simulink model "modeldefinitiu4t"  (Simulink 7.4)
settings: Solver=ode45  StartTime=t0  StopTime=t1  MaxStep=1e-4
values from neighbouring files (symbols this model uses):
  Ap = 90e3*sqrt(2)/sqrt(3)    [parametres.m]
  E0 = 145e3    (= 145000)    [parametres.m]
  f = 50    [parametres.m]
  ida3 = 0    [parametres.m]
  ida4 = 0    [parametres.m]
  it = [0 0.2 0.200001 0.35 0.3500001 t1]    [parametres.m]
  iv = [0 0 100e6 100e6 0 0]    [parametres.m]
  K3 = 1/20    (= 0.05)    [parametres.m]
  K4 = K3    (= 0.05)    [parametres.m]
  Ki = rl/tau    (= 1140.8)    [parametres.m]
  Kp = Ll/tau    (= 93)    [parametres.m]
  L1 = 0.005    [parametres.m]
  L2 = 0.0025    [parametres.m]
  L3 = 0.004    [parametres.m]
  Lac = 30e-3    (= 0.03)    [parametres.m]
  Ll = Lac    (= 0.03)    [parametres.m]
  Lx = 0.052*0.669    (= 0.034788)    [parametres.m]
  R1 = 0.5    [parametres.m]
  R2 = 0.25    [parametres.m]
  R3 = 0.4    [parametres.m]
  Rac = 3.68/10    (= 0.368)    [parametres.m]
  Rx = 4.8*0.669    (= 3.2112)    [parametres.m]
  sc = 0    [parametres.m]
  T = 1/12e3    (= 8.33333333333e-05)    [parametres.m]
undefined symbols (not defined in the file or in its folder): DiscIntNeverNeededParam
libraries: powerlib x62
(part 2 of 2)

== system modeldefinitiu4t/Subsystem5/Càlcul de consignes ==
  note: P
  vzq3 : Inport
  E3 : Inport  Port=2
  Constant : Constant  Value=E0  OutDataType=fixdt(1, 16)  OutScaling=2^0
  Divide1 : Product  Inputs=*/  OutDataType=fixdt(1, 16)  OutScaling=2^-10
  Gain : Gain  Gain=K3  ParameterDataType=fixdt(1, 16)  ParameterScaling=2^0  OutDataType=fixdt(1, 16)  OutScaling=2^0
  Gain1 : Gain  Gain=2/3  ParameterDataType=fixdt(1, 16)  ParameterScaling=2^0  OutDataType=fixdt(1, 16)  OutScaling=2^0
  Gain2 : Gain  ParameterDataType=fixdt(1, 16)  ParameterScaling=2^0  OutDataType=fixdt(1, 16)  OutScaling=2^0  SampleTime=T
  Gain6 : Gain  ParameterDataType=fixdt(1, 16)  ParameterScaling=2^0  OutDataType=fixdt(1, 16)  OutScaling=2^0  SampleTime=T
  Gain7 : Gain  ParameterDataType=fixdt(1, 16)  ParameterScaling=2^0  OutDataType=fixdt(1, 16)  OutScaling=2^0  SampleTime=T
  Product : Product  OutDataType=fixdt(1, 16)  OutScaling=2^0  RndMeth=Zero
  Sum : Sum  Inputs=|+-  OutDataType=fixdt(1, 16)  OutScaling=2^0
  To Workspace3 : ToWorkspace  VariableName=Eref  SampleTime=-1  SaveFormat=Array
  iqa3 : Outport
  wires:
  Constant/1 -> Gain7/1
  Sum/1 -> Gain/1
  Product/1 -> Gain1/1
  Gain/1 -> Product/2
  Gain6/1 -> Sum/1, Product/1
  Gain7/1 -> Sum/2, To Workspace3/1
  Gain1/1 -> Divide1/1  "P"
  vzq3/1 -> Gain2/1
  Divide1/1 -> iqa3/1  "iq*"
  E3/1 -> Gain6/1
  Gain2/1 -> Divide1/2

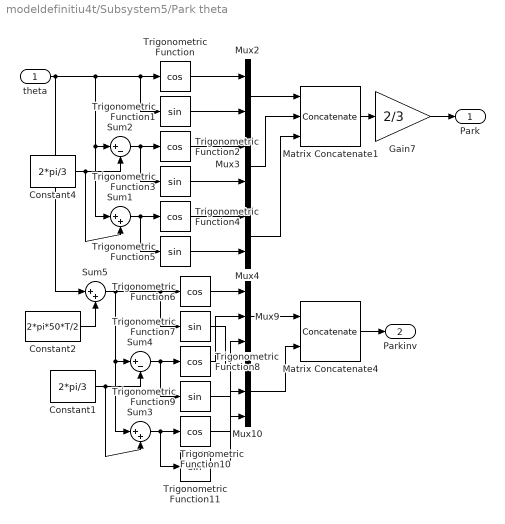
== system modeldefinitiu4t/Subsystem5/Park theta ==
  theta : Inport  PortDimensions=1  OutDataType=sfix(16)  OutScaling=2^0
  Constant1 : Constant  Value=2*pi/3  OutDataType=sfix(16)  OutScaling=2^0  SampleTime=T
  Constant2 : Constant  Value=2*pi*50*T/2  OutDataType=sfix(16)  OutScaling=2^0  SampleTime=T
  Constant4 : Constant  Value=2*pi/3  OutDataType=sfix(16)  OutScaling=2^0  SampleTime=T
  Gain7 : Gain  Gain=2/3  ParameterDataType=sfix(16)  ParameterScaling=2^0  OutDataType=sfix(16)  OutScaling=2^0
  Matrix Concatenate1 : Concatenate  NumInputs=3  Mode=Multidimensional array  ConcatenateDimension=2
  Matrix Concatenate4 : Concatenate  Mode=Multidimensional array  ConcatenateDimension=2
  Mux10 : Mux  Inputs=3
  Mux2 : Mux  Inputs=2
  Mux3 : Mux  Inputs=2
  Mux4 : Mux  Inputs=2
  Mux9 : Mux  Inputs=3
  Sum1 : Sum  Inputs=|++  OutDataType=sfix(16)  OutScaling=2^0
  Sum2 : Sum  Inputs=|+-  OutDataType=sfix(16)  OutScaling=2^0
  Sum3 : Sum  Inputs=|++  OutDataType=sfix(16)  OutScaling=2^0
  Sum4 : Sum  Inputs=|+-  OutDataType=sfix(16)  OutScaling=2^0
  Sum5 : Sum  Inputs=|++  OutDataType=sfix(16)  OutScaling=2^0
  Trigonometric Function{,2,4,6,8,10} (6 alike) : Trigonometry  Operator=cos
  Trigonometric Function{1,3,5,7,9,11} (6 alike) : Trigonometry
  Park : Outport  OutDataType=sfix(16)  OutScaling=2^0
  Parkinv : Outport  Port=2  OutDataType=sfix(16)  OutScaling=2^0
  wires:
  theta/1 -> Sum1/1, Sum2/1, Trigonometric Function/1, Trigonometric Function1/1, Sum5/1
  Sum2/1 -> Trigonometric Function2/1, Trigonometric Function3/1
  Sum1/1 -> Trigonometric Function4/1, Trigonometric Function5/1
  Constant4/1 -> Sum2/2, Sum1/2
  Trigonometric Function/1 -> Mux2/1
  Trigonometric Function1/1 -> Mux2/2
  Trigonometric Function2/1 -> Mux3/1
  Trigonometric Function3/1 -> Mux3/2
  Trigonometric Function4/1 -> Mux4/1
  Trigonometric Function5/1 -> Mux4/2
  Mux2/1 -> Matrix Concatenate1/1
  Mux3/1 -> Matrix Concatenate1/2
  Mux4/1 -> Matrix Concatenate1/3
  Matrix Concatenate1/1 -> Gain7/1
  Gain7/1 -> Park/1
  Sum5/1 -> Trigonometric Function7/1, Trigonometric Function6/1, Sum4/1, Sum3/1
  Sum4/1 -> Trigonometric Function9/1, Trigonometric Function8/1
  Sum3/1 -> Trigonometric Function11/1, Trigonometric Function10/1
  Constant1/1 -> Sum3/2, Sum4/2
  Trigonometric Function6/1 -> Mux9/1
  Trigonometric Function7/1 -> Mux10/1
  Trigonometric Function8/1 -> Mux9/2
  Trigonometric Function9/1 -> Mux10/2
  Trigonometric Function10/1 -> Mux9/3
  Trigonometric Function11/1 -> Mux10/3
  Mux9/1 -> Matrix Concatenate4/1
  Mux10/1 -> Matrix Concatenate4/2
  Matrix Concatenate4/1 -> Parkinv/1
  Constant2/1 -> Sum5/2

== system modeldefinitiu4t/Subsystem5/Subsystem ==
  omega : Inport
  ilqd : Inport  Port=2
  Demux2 : Demux  Outputs=2
  Gain2 : Gain  Gain=Ll  ParameterDataType=sfix(16)  ParameterScaling=2^0  OutDataType=sfix(16)  OutScaling=2^0  SampleTime=T
  Gain3 : Gain  Gain=-Ll  ParameterDataType=sfix(16)  ParameterScaling=2^0  OutDataType=sfix(16)  OutScaling=2^0  SampleTime=T
  Mux1 : Mux  Inputs=2
  Product : Product  OutDataType=fixdt(1, 16)  OutScaling=2^0  RndMeth=Zero
  Product3 : Product  OutDataType=fixdt(1, 16)  OutScaling=2^0  RndMeth=Zero
  desacoblqd1 : Outport
  wires:
  Gain2/1 -> Product3/2
  Gain3/1 -> Product/1
  omega/1 -> Product3/1, Product/2
  ilqd/1 -> Demux2/1
  Demux2/2 -> Gain2/1
  Demux2/1 -> Gain3/1
  Product3/1 -> Mux1/1
  Product/1 -> Mux1/2
  Mux1/1 -> desacoblqd1/1

== system modeldefinitiu4t/Subsystem5/Transformades ==
  In1 : Inport
  Vzabc3 : Inport  Port=2
  Iabc3 : Inport  Port=3
  Gain2 : Gain  ParameterDataType=sfix(16)  ParameterScaling=2^0  OutDataType=sfix(16)  OutScaling=2^0  SampleTime=T
  Gain3 : Gain  ParameterDataType=sfix(16)  ParameterScaling=2^0  OutDataType=sfix(16)  OutScaling=2^0  SampleTime=T
  Gain4 : Gain  ParameterDataType=sfix(16)  ParameterScaling=2^0  OutDataType=sfix(16)  OutScaling=2^0  SampleTime=T
  Product1 : Product  Multiplication=Matrix(*)  OutDataType=sfix(16)  OutScaling=2^0  RndMeth=Zero
  Product2 : Product  Multiplication=Matrix(*)  OutDataType=sfix(16)  OutScaling=2^0  RndMeth=Zero
  To Workspace1 : ToWorkspace  VariableName=Ilabc3  SampleTime=-1  SaveFormat=Array
  To Workspace2 : ToWorkspace  VariableName=Vzabc3  SampleTime=-1  SaveFormat=Array
  Vzqd : Outport
  Iqd : Outport  Port=2
  wires:
  Vzabc3/1 -> Product1/2, To Workspace2/1
  Iabc3/1 -> Product2/2, To Workspace1/1
  Product1/1 -> Gain2/1
  Gain4/1 -> Product1/1, Product2/1
  Product2/1 -> Gain3/1
  In1/1 -> Gain4/1
  Gain2/1 -> Vzqd/1
  Gain3/1 -> Iqd/1
